simulink library "dsrc_transmitter"  (Simulink 8.2)
settings: Solver=ode1  StartTime=0.0  StopTime=Inf  FixedStep=0.001  RelTol=1e-3
PostLoadFcn:
  | , if any(exist('dsrtsu_mdlpostloadfcn', 'file') == [2, 3, 6]), try dsrtsu_mdlpostloadfcn('Execute', bdroot); catch fprintf('Error in PostLoadFcn (dsrtsu_mdlpostloadfcn) for model "%s":\n %s\n', bdroot, lasterr); end, end,
libraries: simulink x10, rtitttasklib x2, rtiethernetudplib x1, parse_utils x1
(part 1 of 2)
settings Model: DSRTSU_INTERNAL_RTI_VER=440  DSRTSU_INTERNAL_RTI_TYPE=rti1401  DSRTSU_INTERNAL_RTIFPGA=30  Creator=leidos  LastModifiedBy=Admin

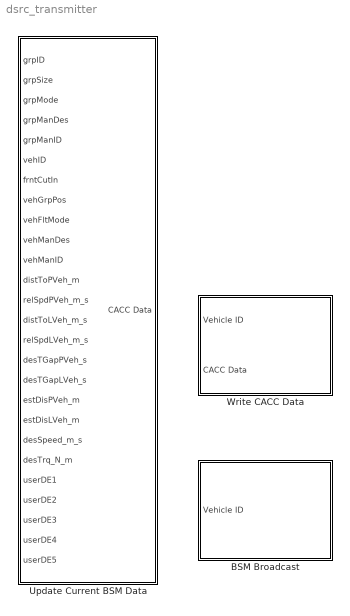
== system dsrc_transmitter ==
  BSM Broadcast : Subsystem
  Update Current BSM Data : Subsystem
  Write CACC Data : Subsystem

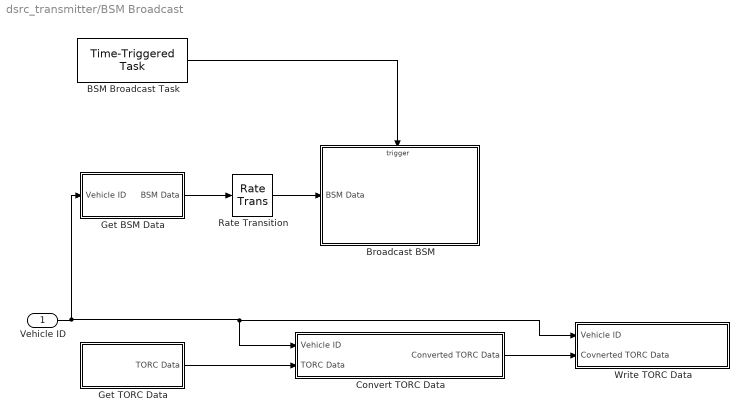
== system dsrc_transmitter/BSM Broadcast ==
  Vehicle ID : Inport
  BSM Broadcast Task : rtitttasklib/Time-Triggered Task  TimeTriggerId=BSM_TX  TLCFileName=rtitimetriggeredtask  DSProperties=struct('RTI',struct('Version',uint32(1),'BlockType',struct('isSLSource',uint8(1),'isSLSink',uint8(0),'isHWSource',uint8(0),'isHWSink',uint8(0),'isSetup',uint8(0),'isInline',uint8(1),'isNonInline',uint8(0),'isInterrupt',uint8(0),'isChannelwise',uint8(0)),'IOBoardType','RTITIMETRIGGER','UnitType','TIMETRIGGERED','Identifier','TASK','DialogType','SL','BlockSet','NONE','SlaveProcessor','NONE'))  RTIBlockInterface=struct('OutputPortsActive',1,'OutputPortsWidth',int32(1),'FunctionCall',uint32(0),'OutputPortsName',{{[' ']}},'InitLevel',3,'BlockDisplay',{{['Time-Triggered Task\nID: ''''BSM_TX'''''],'center'}},'IconTransparency','off','BlockName',struct('Token',{{['Time-Triggered Task']}}),'MaskDescription',['Specifies a time-triggered task. The task trigger times are set by the assigned Time-Trigger Set block.' char(10) '' char(10) 'This block can only be used together with the Time-Trigger Set block.'])  RTIBlockParameters=struct('TimeTriggerId',{{'BSM_TX','OFF',[]}},'TLCFileName',{{'rtitimetriggeredtask','OFF',[]}})  RTISFcnParameters=struct('TLCFileName','char')  RTIBlockParaDefault=struct('TimeTriggerId','TT_ID','TLCFileName','rtitimetriggeredtask')
  Broadcast BSM : Subsystem
  Convert TORC Data : Subsystem
  Get BSM Data : Subsystem
  Get TORC Data : Subsystem
  Rate Transition : RateTransition  Deterministic=off
  Write TORC Data : Subsystem
  wires:
  Get BSM Data/1(BSM Data) -> Rate Transition/1
  BSM Broadcast Task/1 -> Broadcast BSM/Trigger
  Get TORC Data/1(TORC Data) -> Convert TORC Data/2(TORC Data)
  Convert TORC Data/1(Converted TORC Data) -> Write TORC Data/2(Covnerted TORC Data)
  Vehicle ID/1 -> Write TORC Data/1(Vehicle ID), Convert TORC Data/1(Vehicle ID), Get BSM Data/1(Vehicle ID)
  Rate Transition/1 -> Broadcast BSM/1(BSM Data)

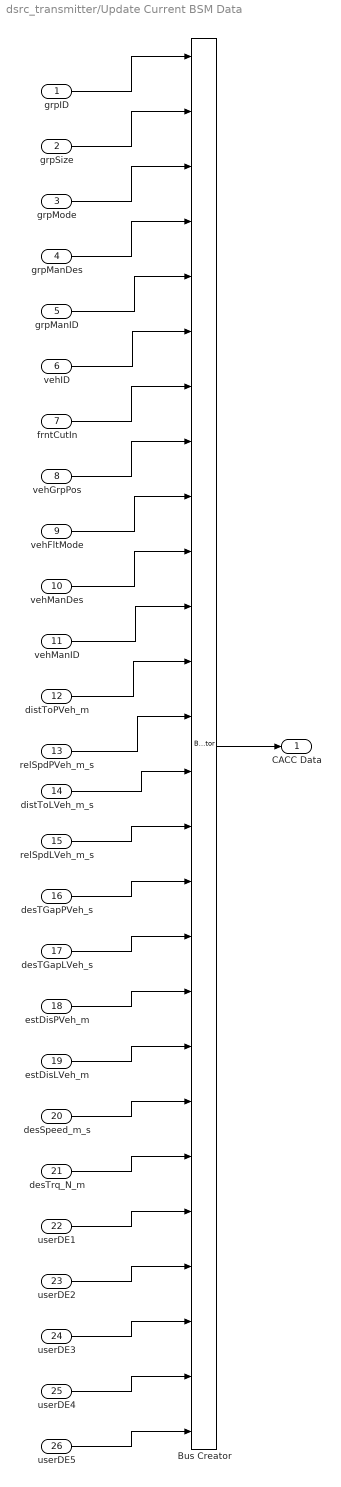
== system dsrc_transmitter/Update Current BSM Data ==
  grpID : Inport
  grpSize : Inport  Port=2
  grpMode : Inport  Port=3
  grpManDes : Inport  Port=4
  grpManID : Inport  Port=5
  vehID : Inport  Port=6
  frntCutIn : Inport  Port=7
  vehGrpPos : Inport  Port=8
  vehFltMode : Inport  Port=9
  vehManDes : Inport  Port=10
  vehManID : Inport  Port=11
  distToPVeh_m : Inport  Port=12
  relSpdPVeh_m_s : Inport  Port=13
  distToLVeh_m_s : Inport  Port=14
  relSpdLVeh_m_s : Inport  Port=15
  desTGapPVeh_s : Inport  Port=16
  desTGapLVeh_s : Inport  Port=17
  estDisPVeh_m : Inport  Port=18
  estDisLVeh_m : Inport  Port=19
  desSpeed_m_s : Inport  Port=20
  desTrq_N_m : Inport  Port=21
  userDE1 : Inport  Port=22
  userDE2 : Inport  Port=23
  userDE3 : Inport  Port=24
  userDE4 : Inport  Port=25
  userDE5 : Inport  Port=26
  Bus Creator : BusCreator  Inputs=26
  CACC Data : Outport
  wires:
  grpID/1 -> Bus Creator/1
  grpSize/1 -> Bus Creator/2
  grpMode/1 -> Bus Creator/3
  grpManDes/1 -> Bus Creator/4
  grpManID/1 -> Bus Creator/5
  vehID/1 -> Bus Creator/6
  frntCutIn/1 -> Bus Creator/7
  vehGrpPos/1 -> Bus Creator/8
  vehFltMode/1 -> Bus Creator/9
  vehManDes/1 -> Bus Creator/10
  vehManID/1 -> Bus Creator/11
  distToPVeh_m/1 -> Bus Creator/12
  relSpdPVeh_m_s/1 -> Bus Creator/13
  distToLVeh_m_s/1 -> Bus Creator/14
  relSpdLVeh_m_s/1 -> Bus Creator/15
  desTGapPVeh_s/1 -> Bus Creator/16
  desTGapLVeh_s/1 -> Bus Creator/17
  estDisPVeh_m/1 -> Bus Creator/18
  estDisLVeh_m/1 -> Bus Creator/19
  desSpeed_m_s/1 -> Bus Creator/20
  desTrq_N_m/1 -> Bus Creator/21
  userDE1/1 -> Bus Creator/22
  userDE2/1 -> Bus Creator/23
  userDE3/1 -> Bus Creator/24
  userDE4/1 -> Bus Creator/25
  userDE5/1 -> Bus Creator/26
  Bus Creator/1 -> CACC Data/1

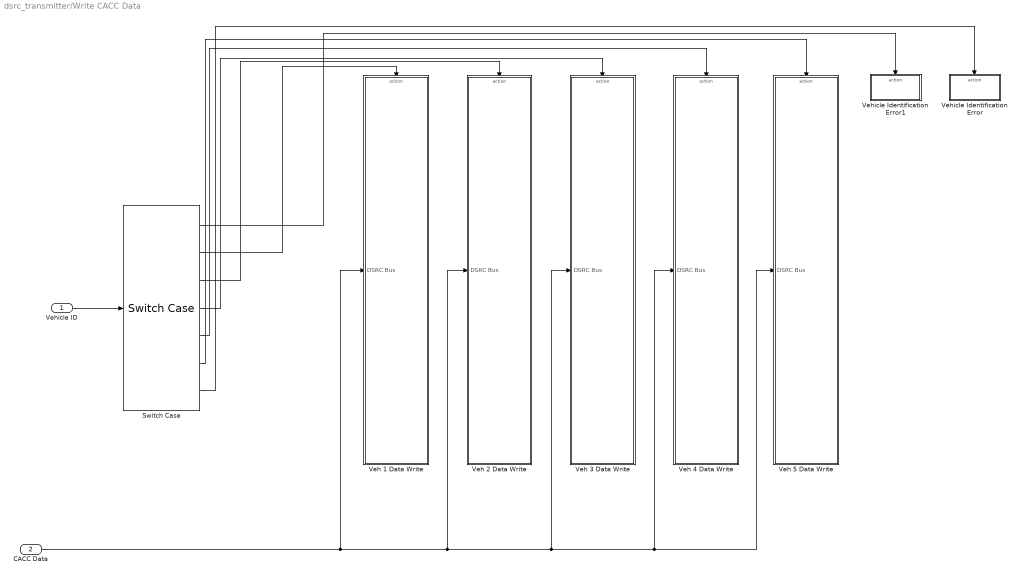
== system dsrc_transmitter/Write CACC Data ==
  Vehicle ID : Inport
  CACC Data : Inport  Port=2
  Switch Case : SwitchCase  CaseConditions={0,96,97,98,99,100}
  Veh 1 Data Write : Subsystem  TreatAsAtomicUnit=on
  Veh 2 Data Write : Subsystem  TreatAsAtomicUnit=on
  Veh 3 Data Write : Subsystem  TreatAsAtomicUnit=on
  Veh 4 Data Write : Subsystem  TreatAsAtomicUnit=on
  Veh 5 Data Write : Subsystem  TreatAsAtomicUnit=on
  Vehicle Identification Error : Subsystem  TreatAsAtomicUnit=on
  Vehicle Identification Error1 : Subsystem  TreatAsAtomicUnit=on
  wires:
  CACC Data/1 -> Veh 5 Data Write/1(DSRC Bus), Veh 4 Data Write/1(DSRC Bus), Veh 3 Data Write/1(DSRC Bus), Veh 2 Data Write/1(DSRC Bus), Veh 1 Data Write/1(DSRC Bus)
  Switch Case/2 -> Veh 1 Data Write/Action
  Switch Case/3 -> Veh 2 Data Write/Action
  Switch Case/4 -> Veh 3 Data Write/Action
  Switch Case/5 -> Veh 4 Data Write/Action
  Switch Case/6 -> Veh 5 Data Write/Action
  Switch Case/1 -> Vehicle Identification Error1/Action
  Switch Case/7 -> Vehicle Identification Error/Action
  Vehicle ID/1 -> Switch Case/1

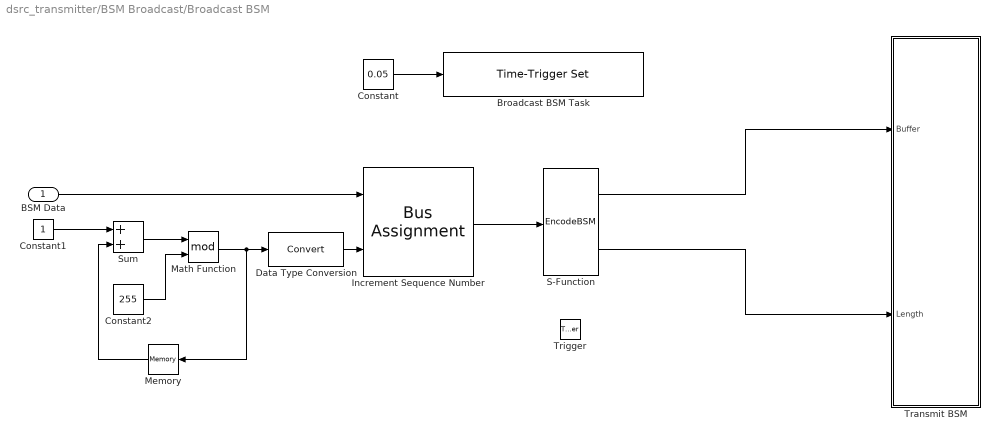
== system dsrc_transmitter/BSM Broadcast/Broadcast BSM ==
  BSM Data : Inport
  Trigger : TriggerPort  TriggerType=function-call  PortDimensions=1
  Broadcast BSM Task : rtitttasklib/Time-Trigger Set  TimeTriggerId=BSM_TX  SampleTime=-1  RegisterAtSimulationStart=on  TLCFileName=rtitimetriggerset  DSProperties=struct('RTI',struct('Version',uint32(1),'BlockType',struct('isSLSource',uint8(1),'isSLSink',uint8(0),'isHWSource',uint8(0),'isHWSink',uint8(0),'isSetup',uint8(0),'isInline',uint8(1),'isNonInline',uint8(0),'isInterrupt',uint8(0),'isChannelwise',uint8(0)),'IOBoardType','RTITIMETRIGGER','UnitType','TIMETRIGGERED','Identifier','SET','DialogType','SL','BlockSet','NONE','SlaveProcessor','NONE'))  RTIBlockInterface=struct('InputPortsActive',1,'InputPortsWidth',{{'DYNAMICALLY_SIZED'}},'InputPortsDataType',{{'SS_DOUBLE'}},'InputPortsName',{{['Trigger delay']}},'InitLevel',3,'BlockDisplay',{{['Time-Trigger Set\nID: ''''BSM_TX'''''],'center'}},'IconTransparency','on','BlockName',struct('Token',{{['Time-Trigger Set']}}),'MaskDescription',['When this block is evaluated it sets the task trigger times for the assigned time-triggered task.' char(10) '' char(10) 'This block can only be used together with the Time-Triggered Task block.'],'SampleTime',{{-1}})  RTIBlockParameters=struct('TimeTriggerId',{{'BSM_TX','OFF',[]}},'SampleTime',{{-1,'OFF',[]}},'RegisterAtSimulationStart',{{logical(1),'OFF',[]}},'TLCFileName',{{'rtitimetriggerset','OFF',[]}})  RTISFcnParameters=struct('TimeTriggerId','char','SampleTime','double','TLCFileName','char','RegisterAtSimulationStart','double')  RTIBlockParaDefault=struct('TimeTriggerId','TT_ID','SampleTime',-1,'RegisterAtSimulationStart',0,'TLCFileName','rtitimetriggerset')
  Constant : Constant  Value=0.05
  Constant1 : Constant
  Constant2 : Constant  Value=255
  Data Type Conversion : DataTypeConversion
  Increment Sequence Number : BusAssignment  AssignedSignals=msgCnt
  Math Function : Math  Operator=mod  SaturateOnIntegerOverflow=on
  Memory : Memory  InheritSampleTime=on
  S-Function : S-Function  FunctionName=EncodeBSM  SFunctionModules='EncodeBSM_wrapper bsm_encoder der_encoder'  EnableBusSupport=off
  Sum : Sum  SaturateOnIntegerOverflow=on  InputSameDT=on  OutDataTypeStr=Inherit: Same as first input
  Transmit BSM : Subsystem
  wires:
  S-Function/1 -> Transmit BSM/1(Buffer)
  S-Function/2 -> Transmit BSM/2(Length)
  BSM Data/1 -> Increment Sequence Number/1
  Constant/1 -> Broadcast BSM Task/1
  Constant1/1 -> Sum/1
  Memory/1 -> Sum/2
  Sum/1 -> Math Function/1
  Increment Sequence Number/1 -> S-Function/1
  Math Function/1 -> Memory/1, Data Type Conversion/1
  Constant2/1 -> Math Function/2
  Data Type Conversion/1 -> Increment Sequence Number/2

== system dsrc_transmitter/BSM Broadcast/Convert TORC Data ==
  Vehicle ID : Inport
  TORC Data : Inport  Port=2
  Data Conversion : Subsystem
  Data Type Conversion : DataTypeConversion
  Converted TORC Data : Outport
  wires:
  TORC Data/1 -> Data Conversion/2(TORC Data)
  Data Conversion/1(BSM Data) -> Converted TORC Data/1
  Vehicle ID/1 -> Data Type Conversion/1
  Data Type Conversion/1 -> Data Conversion/1(Vehicle ID)

== system dsrc_transmitter/BSM Broadcast/Get BSM Data ==
  Vehicle ID : Inport
  BSM Data Read : Subsystem
  BSM Data : Outport
  wires:
  BSM Data Read/1(Cur Veh BSM Data) -> BSM Data/1
  Vehicle ID/1 -> BSM Data Read/1(Veh ID)

== system dsrc_transmitter/BSM Broadcast/Get TORC Data ==
  Bus Creator : BusCreator  Inputs=28
  Data Store Read : DataStoreRead  DataStoreName=CarmaData  DataStoreElements=CarmaData.acc_status#CarmaData.requested_cacc_state#CarmaData.radar_status#CarmaData.throttle_pedal_deflect_percent#CarmaData.acc_set_speed_m_s#CarmaData.local_north_m#CarmaData.local_east_m#CarmaData.local_down_m#CarmaData.global_roll_deg#CarmaData.global_pitch_deg#CarmaData.global_yaw_deg#CarmaData.horizontal_pos_accuracy_m#CarmaData.vertical_pos_accuracy_m#CarmaData.velocity_fwd_m_s#CarmaData.velocity_right_m_s#CarmaData.velocity_down_m_s#CarmaData.velocity_accuracy_m_s#CarmaData.accel_m_s2#CarmaData.accel_right_m_s2#CarmaData.accel_down_m_s2#CarmaData.speed_m_s#CarmaData.steering_wheel_angle_deg#CarmaData.brk_light_flag#CarmaData.global_utc_time_s#CarmaData.global_lat_deg#CarmaData.global_long_deg#CarmaData.global_alt_m#CarmaData.path_ctrl_status.value
  TORC Data : Outport
  wires:
  Data Store Read/1 -> Bus Creator/1
  Data Store Read/2 -> Bus Creator/2
  Data Store Read/3 -> Bus Creator/3
  Data Store Read/4 -> Bus Creator/4
  Data Store Read/5 -> Bus Creator/5
  Data Store Read/6 -> Bus Creator/6
  Data Store Read/7 -> Bus Creator/7
  Data Store Read/8 -> Bus Creator/8
  Data Store Read/9 -> Bus Creator/9
  Data Store Read/10 -> Bus Creator/10
  Data Store Read/12 -> Bus Creator/12
  Data Store Read/13 -> Bus Creator/13
  Data Store Read/14 -> Bus Creator/14
  Data Store Read/15 -> Bus Creator/15
  Data Store Read/16 -> Bus Creator/16
  Data Store Read/17 -> Bus Creator/17
  Data Store Read/18 -> Bus Creator/18
  Data Store Read/19 -> Bus Creator/19
  Data Store Read/20 -> Bus Creator/20
  Data Store Read/21 -> Bus Creator/21
  Data Store Read/22 -> Bus Creator/22
  Data Store Read/23 -> Bus Creator/23
  Data Store Read/11 -> Bus Creator/11
  Bus Creator/1 -> TORC Data/1
  Data Store Read/24 -> Bus Creator/24
  Data Store Read/25 -> Bus Creator/25
  Data Store Read/26 -> Bus Creator/26
  Data Store Read/27 -> Bus Creator/27
  Data Store Read/28 -> Bus Creator/28

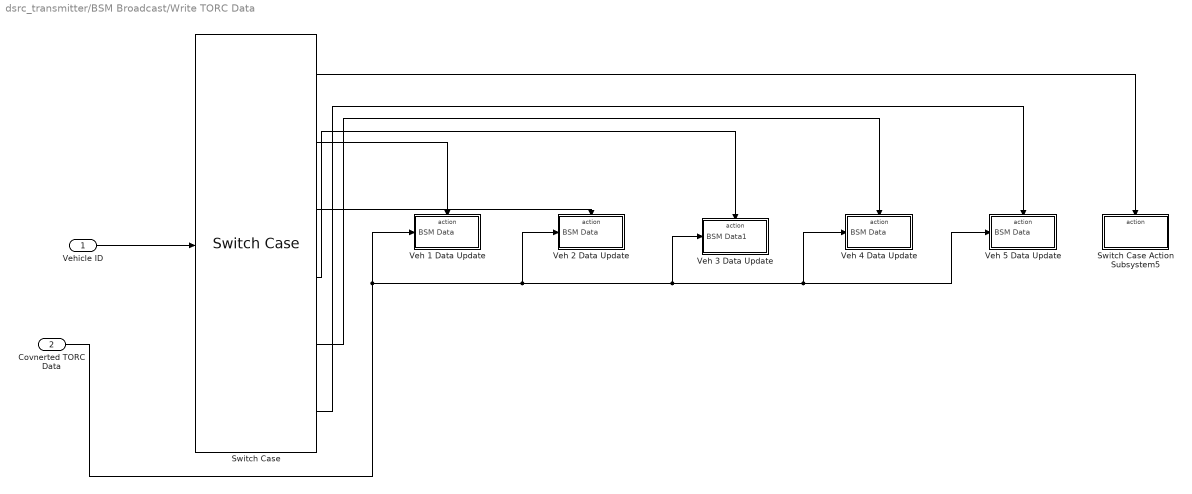
== system dsrc_transmitter/BSM Broadcast/Write TORC Data ==
  Vehicle ID : Inport
  Covnerted TORC Data : Inport  Port=2
  Switch Case : SwitchCase  CaseConditions={0,96,97,98,99,100}  ShowDefaultCase=off
  Switch Case Action Subsystem5 : Subsystem  TreatAsAtomicUnit=on
  Veh 1 Data Update : Subsystem  TreatAsAtomicUnit=on
  Veh 2 Data Update : Subsystem  TreatAsAtomicUnit=on
  Veh 3 Data Update : Subsystem  TreatAsAtomicUnit=on
  Veh 4 Data Update : Subsystem  TreatAsAtomicUnit=on
  Veh 5 Data Update : Subsystem  TreatAsAtomicUnit=on
  wires:
  Switch Case/2 -> Veh 1 Data Update/Action
  Switch Case/3 -> Veh 2 Data Update/Action
  Switch Case/4 -> Veh 3 Data Update/Action
  Switch Case/5 -> Veh 4 Data Update/Action
  Switch Case/6 -> Veh 5 Data Update/Action
  Switch Case/1 -> Switch Case Action Subsystem5/Action
  Covnerted TORC Data/1 -> Veh 1 Data Update/1(BSM Data), Veh 2 Data Update/1(BSM Data), Veh 3 Data Update/1(BSM Data1), Veh 5 Data Update/1(BSM Data), Veh 4 Data Update/1(BSM Data)
  Vehicle ID/1 -> Switch Case/1

== system dsrc_transmitter/Write CACC Data/Veh 1 Data Write ==
  DSRC Bus : Inport
  Action Port : ActionPort
  Bus Selector : BusSelector  OutputSignals=signal1,signal2,signal3,signal4,signal5,signal6,signal7,signal8,signal9,signal10,signal11,signal12,signal13,signal14,signal15,signal16,signal17,signal18,signal19,signal20,signal21,signal22,signal23,signal24,signal25,signal26
  Data Store Write : DataStoreWrite  DataStoreName=BSMStoreSignal  DataStoreElements=BSMStoreSignal.Veh1BSM.grpID#BSMStoreSignal.Veh1BSM.grpSize#BSMStoreSignal.Veh1BSM.grpMode#BSMStoreSignal.Veh1BSM.grpManDes#BSMStoreSignal.Veh1BSM.grpManID#BSMStoreSignal.Veh1BSM.vehID#BSMStoreSignal.Veh1BSM.frntCutIn#BSMStoreSignal.Veh1BSM.vehGrpPos#BSMStoreSignal.Veh1BSM.vehFltMode#BSMStoreSignal.Veh1BSM.vehManDes#BSMStoreSignal.Veh1BSM.vehManID#BSMStoreSignal.Veh1BSM.distToPVeh_m#BSMStoreSignal.Veh1BSM.relSpdPVeh_m_s#BSMStoreSignal.Veh1BSM.distToLVeh_m#BSMStoreSignal.Veh1BSM.relSpdLVeh_m_s#BSMStoreSignal.Veh1BSM.desTGapPVeh_s#BSMStoreSignal.Veh1BSM.desTGapLVeh_s#BSMStoreSignal.Veh1BSM.estDisPVeh_m#BSMStoreSignal.Veh1BSM.estDisLVeh_m#BSMStoreSignal.Veh1BSM.desSpeed_m_s#BSMStoreSignal.Veh1BSM.desTrq_N_m#BSMStoreSignal.Veh1BSM.userDE1#BSMStoreSignal.Veh1BSM.userDE2#BSMStoreSignal.Veh1BSM.userDE3#BSMStoreSignal.Veh1BSM.userDE4#BSMStoreSignal.Veh1BSM.userDE5
  wires:
  DSRC Bus/1 -> Bus Selector/1
  Bus Selector/1 -> Data Store Write/1  "<signal1>"
  Bus Selector/2 -> Data Store Write/2  "<signal2>"
  Bus Selector/3 -> Data Store Write/3  "<signal3>"
  Bus Selector/4 -> Data Store Write/4  "<signal4>"
  Bus Selector/5 -> Data Store Write/5  "<signal5>"
  Bus Selector/6 -> Data Store Write/6  "<signal6>"
  Bus Selector/7 -> Data Store Write/7  "<signal7>"
  Bus Selector/8 -> Data Store Write/8  "<signal8>"
  Bus Selector/9 -> Data Store Write/9  "<signal9>"
  Bus Selector/10 -> Data Store Write/10  "<signal10>"
  Bus Selector/11 -> Data Store Write/11  "<signal11>"
  Bus Selector/12 -> Data Store Write/12  "<signal12>"
  Bus Selector/13 -> Data Store Write/13  "<signal13>"
  Bus Selector/14 -> Data Store Write/14  "<signal14>"
  Bus Selector/15 -> Data Store Write/15  "<signal15>"
  Bus Selector/16 -> Data Store Write/16  "<signal16>"
  Bus Selector/17 -> Data Store Write/17  "<signal17>"
  Bus Selector/18 -> Data Store Write/18  "<signal18>"
  Bus Selector/19 -> Data Store Write/19  "<signal19>"
  Bus Selector/20 -> Data Store Write/20  "<signal20>"
  Bus Selector/21 -> Data Store Write/21  "<signal21>"
  Bus Selector/22 -> Data Store Write/22  "<signal22>"
  Bus Selector/23 -> Data Store Write/23  "<signal23>"
  Bus Selector/24 -> Data Store Write/24  "<signal24>"
  Bus Selector/25 -> Data Store Write/25  "<signal25>"
  Bus Selector/26 -> Data Store Write/26  "<signal26>"

== system dsrc_transmitter/Write CACC Data/Veh 2 Data Write ==
  DSRC Bus : Inport
  Action Port : ActionPort
  Bus Selector : BusSelector  OutputSignals=signal1,signal2,signal3,signal4,signal5,signal6,signal7,signal8,signal9,signal10,signal11,signal12,signal13,signal14,signal15,signal16,signal17,signal18,signal19,signal20,signal21,signal22,signal23,signal24,signal25,signal26
  Data Store Write : DataStoreWrite  DataStoreName=BSMStoreSignal  DataStoreElements=BSMStoreSignal.Veh2BSM.grpID#BSMStoreSignal.Veh2BSM.grpSize#BSMStoreSignal.Veh2BSM.grpMode#BSMStoreSignal.Veh2BSM.grpManDes#BSMStoreSignal.Veh2BSM.grpManID#BSMStoreSignal.Veh2BSM.vehID#BSMStoreSignal.Veh2BSM.frntCutIn#BSMStoreSignal.Veh2BSM.vehGrpPos#BSMStoreSignal.Veh2BSM.vehFltMode#BSMStoreSignal.Veh2BSM.vehManDes#BSMStoreSignal.Veh2BSM.vehManID#BSMStoreSignal.Veh2BSM.distToPVeh_m#BSMStoreSignal.Veh2BSM.relSpdPVeh_m_s#BSMStoreSignal.Veh2BSM.distToLVeh_m#BSMStoreSignal.Veh2BSM.relSpdLVeh_m_s#BSMStoreSignal.Veh2BSM.desTGapPVeh_s#BSMStoreSignal.Veh2BSM.desTGapLVeh_s#BSMStoreSignal.Veh2BSM.estDisPVeh_m#BSMStoreSignal.Veh2BSM.estDisLVeh_m#BSMStoreSignal.Veh2BSM.desSpeed_m_s#BSMStoreSignal.Veh2BSM.desTrq_N_m#BSMStoreSignal.Veh2BSM.userDE1#BSMStoreSignal.Veh2BSM.userDE2#BSMStoreSignal.Veh2BSM.userDE3#BSMStoreSignal.Veh2BSM.userDE4#BSMStoreSignal.Veh2BSM.userDE5
  wires:
  DSRC Bus/1 -> Bus Selector/1
  Bus Selector/1 -> Data Store Write/1  "<signal1>"
  Bus Selector/2 -> Data Store Write/2  "<signal2>"
  Bus Selector/3 -> Data Store Write/3  "<signal3>"
  Bus Selector/4 -> Data Store Write/4  "<signal4>"
  Bus Selector/5 -> Data Store Write/5  "<signal5>"
  Bus Selector/6 -> Data Store Write/6  "<signal6>"
  Bus Selector/7 -> Data Store Write/7  "<signal7>"
  Bus Selector/8 -> Data Store Write/8  "<signal8>"
  Bus Selector/9 -> Data Store Write/9  "<signal9>"
  Bus Selector/10 -> Data Store Write/10  "<signal10>"
  Bus Selector/11 -> Data Store Write/11  "<signal11>"
  Bus Selector/12 -> Data Store Write/12  "<signal12>"
  Bus Selector/13 -> Data Store Write/13  "<signal13>"
  Bus Selector/14 -> Data Store Write/14  "<signal14>"
  Bus Selector/15 -> Data Store Write/15  "<signal15>"
  Bus Selector/16 -> Data Store Write/16  "<signal16>"
  Bus Selector/17 -> Data Store Write/17  "<signal17>"
  Bus Selector/18 -> Data Store Write/18  "<signal18>"
  Bus Selector/19 -> Data Store Write/19  "<signal19>"
  Bus Selector/20 -> Data Store Write/20  "<signal20>"
  Bus Selector/21 -> Data Store Write/21  "<signal21>"
  Bus Selector/22 -> Data Store Write/22  "<signal22>"
  Bus Selector/23 -> Data Store Write/23  "<signal23>"
  Bus Selector/24 -> Data Store Write/24  "<signal24>"
  Bus Selector/25 -> Data Store Write/25  "<signal25>"
  Bus Selector/26 -> Data Store Write/26  "<signal26>"

== system dsrc_transmitter/Write CACC Data/Veh 3 Data Write ==
  DSRC Bus : Inport
  Action Port : ActionPort
  Bus Selector : BusSelector  OutputSignals=signal1,signal2,signal3,signal4,signal5,signal6,signal7,signal8,signal9,signal10,signal11,signal12,signal13,signal14,signal15,signal16,signal17,signal18,signal19,signal20,signal21,signal22,signal23,signal24,signal25,signal26
  Data Store Write : DataStoreWrite  DataStoreName=BSMStoreSignal  DataStoreElements=BSMStoreSignal.Veh3BSM.grpID#BSMStoreSignal.Veh3BSM.grpSize#BSMStoreSignal.Veh3BSM.grpMode#BSMStoreSignal.Veh3BSM.grpManDes#BSMStoreSignal.Veh3BSM.grpManID#BSMStoreSignal.Veh3BSM.vehID#BSMStoreSignal.Veh3BSM.frntCutIn#BSMStoreSignal.Veh3BSM.vehGrpPos#BSMStoreSignal.Veh3BSM.vehFltMode#BSMStoreSignal.Veh3BSM.vehManDes#BSMStoreSignal.Veh3BSM.vehManID#BSMStoreSignal.Veh3BSM.distToPVeh_m#BSMStoreSignal.Veh3BSM.relSpdPVeh_m_s#BSMStoreSignal.Veh3BSM.distToLVeh_m#BSMStoreSignal.Veh3BSM.relSpdLVeh_m_s#BSMStoreSignal.Veh3BSM.desTGapPVeh_s#BSMStoreSignal.Veh3BSM.desTGapLVeh_s#BSMStoreSignal.Veh3BSM.estDisPVeh_m#BSMStoreSignal.Veh3BSM.estDisLVeh_m#BSMStoreSignal.Veh3BSM.desSpeed_m_s#BSMStoreSignal.Veh3BSM.desTrq_N_m#BSMStoreSignal.Veh3BSM.userDE1#BSMStoreSignal.Veh3BSM.userDE2#BSMStoreSignal.Veh3BSM.userDE3#BSMStoreSignal.Veh3BSM.userDE4#BSMStoreSignal.Veh3BSM.userDE5
  wires:
  DSRC Bus/1 -> Bus Selector/1
  Bus Selector/1 -> Data Store Write/1  "<signal1>"
  Bus Selector/2 -> Data Store Write/2  "<signal2>"
  Bus Selector/3 -> Data Store Write/3  "<signal3>"
  Bus Selector/4 -> Data Store Write/4  "<signal4>"
  Bus Selector/5 -> Data Store Write/5  "<signal5>"
  Bus Selector/6 -> Data Store Write/6  "<signal6>"
  Bus Selector/7 -> Data Store Write/7  "<signal7>"
  Bus Selector/8 -> Data Store Write/8  "<signal8>"
  Bus Selector/9 -> Data Store Write/9  "<signal9>"
  Bus Selector/10 -> Data Store Write/10  "<signal10>"
  Bus Selector/11 -> Data Store Write/11  "<signal11>"
  Bus Selector/12 -> Data Store Write/12  "<signal12>"
  Bus Selector/13 -> Data Store Write/13  "<signal13>"
  Bus Selector/14 -> Data Store Write/14  "<signal14>"
  Bus Selector/15 -> Data Store Write/15  "<signal15>"
  Bus Selector/16 -> Data Store Write/16  "<signal16>"
  Bus Selector/17 -> Data Store Write/17  "<signal17>"
  Bus Selector/18 -> Data Store Write/18  "<signal18>"
  Bus Selector/19 -> Data Store Write/19  "<signal19>"
  Bus Selector/20 -> Data Store Write/20  "<signal20>"
  Bus Selector/21 -> Data Store Write/21  "<signal21>"
  Bus Selector/22 -> Data Store Write/22  "<signal22>"
  Bus Selector/23 -> Data Store Write/23  "<signal23>"
  Bus Selector/24 -> Data Store Write/24  "<signal24>"
  Bus Selector/25 -> Data Store Write/25  "<signal25>"
  Bus Selector/26 -> Data Store Write/26  "<signal26>"

== system dsrc_transmitter/Write CACC Data/Veh 4 Data Write ==
  DSRC Bus : Inport
  Action Port : ActionPort
  Bus Selector : BusSelector  OutputSignals=signal1,signal2,signal3,signal4,signal5,signal6,signal7,signal8,signal9,signal10,signal11,signal12,signal13,signal14,signal15,signal16,signal17,signal18,signal19,signal20,signal21,signal22,signal23,signal24,signal25,signal26
  Data Store Write : DataStoreWrite  DataStoreName=BSMStoreSignal  DataStoreElements=BSMStoreSignal.Veh4BSM.grpID#BSMStoreSignal.Veh4BSM.grpSize#BSMStoreSignal.Veh4BSM.grpMode#BSMStoreSignal.Veh4BSM.grpManDes#BSMStoreSignal.Veh4BSM.grpManID#BSMStoreSignal.Veh4BSM.vehID#BSMStoreSignal.Veh4BSM.frntCutIn#BSMStoreSignal.Veh4BSM.vehGrpPos#BSMStoreSignal.Veh4BSM.vehFltMode#BSMStoreSignal.Veh4BSM.vehManDes#BSMStoreSignal.Veh4BSM.vehManID#BSMStoreSignal.Veh4BSM.distToPVeh_m#BSMStoreSignal.Veh4BSM.relSpdPVeh_m_s#BSMStoreSignal.Veh4BSM.distToLVeh_m#BSMStoreSignal.Veh4BSM.relSpdLVeh_m_s#BSMStoreSignal.Veh4BSM.desTGapPVeh_s#BSMStoreSignal.Veh4BSM.desTGapLVeh_s#BSMStoreSignal.Veh4BSM.estDisPVeh_m#BSMStoreSignal.Veh4BSM.estDisLVeh_m#BSMStoreSignal.Veh4BSM.desSpeed_m_s#BSMStoreSignal.Veh4BSM.desTrq_N_m#BSMStoreSignal.Veh4BSM.userDE1#BSMStoreSignal.Veh4BSM.userDE2#BSMStoreSignal.Veh4BSM.userDE3#BSMStoreSignal.Veh4BSM.userDE4#BSMStoreSignal.Veh4BSM.userDE5
  wires:
  DSRC Bus/1 -> Bus Selector/1
  Bus Selector/1 -> Data Store Write/1  "<signal1>"
  Bus Selector/2 -> Data Store Write/2  "<signal2>"
  Bus Selector/3 -> Data Store Write/3  "<signal3>"
  Bus Selector/4 -> Data Store Write/4  "<signal4>"
  Bus Selector/5 -> Data Store Write/5  "<signal5>"
  Bus Selector/6 -> Data Store Write/6  "<signal6>"
  Bus Selector/7 -> Data Store Write/7  "<signal7>"
  Bus Selector/8 -> Data Store Write/8  "<signal8>"
  Bus Selector/9 -> Data Store Write/9  "<signal9>"
  Bus Selector/10 -> Data Store Write/10  "<signal10>"
  Bus Selector/11 -> Data Store Write/11  "<signal11>"
  Bus Selector/12 -> Data Store Write/12  "<signal12>"
  Bus Selector/13 -> Data Store Write/13  "<signal13>"
  Bus Selector/14 -> Data Store Write/14  "<signal14>"
  Bus Selector/15 -> Data Store Write/15  "<signal15>"
  Bus Selector/16 -> Data Store Write/16  "<signal16>"
  Bus Selector/17 -> Data Store Write/17  "<signal17>"
  Bus Selector/18 -> Data Store Write/18  "<signal18>"
  Bus Selector/19 -> Data Store Write/19  "<signal19>"
  Bus Selector/20 -> Data Store Write/20  "<signal20>"
  Bus Selector/21 -> Data Store Write/21  "<signal21>"
  Bus Selector/22 -> Data Store Write/22  "<signal22>"
  Bus Selector/23 -> Data Store Write/23  "<signal23>"
  Bus Selector/24 -> Data Store Write/24  "<signal24>"
  Bus Selector/25 -> Data Store Write/25  "<signal25>"
  Bus Selector/26 -> Data Store Write/26  "<signal26>"

== system dsrc_transmitter/Write CACC Data/Veh 5 Data Write ==
  DSRC Bus : Inport
  Action Port : ActionPort
  Bus Selector : BusSelector  OutputSignals=signal1,signal2,signal3,signal4,signal5,signal6,signal7,signal8,signal9,signal10,signal11,signal12,signal13,signal14,signal15,signal16,signal17,signal18,signal19,signal20,signal21,signal22,signal23,signal24,signal25,signal26
  Data Store Write : DataStoreWrite  DataStoreName=BSMStoreSignal  DataStoreElements=BSMStoreSignal.Veh5BSM.grpID#BSMStoreSignal.Veh5BSM.grpSize#BSMStoreSignal.Veh5BSM.grpMode#BSMStoreSignal.Veh5BSM.grpManDes#BSMStoreSignal.Veh5BSM.grpManID#BSMStoreSignal.Veh5BSM.vehID#BSMStoreSignal.Veh5BSM.frntCutIn#BSMStoreSignal.Veh5BSM.vehGrpPos#BSMStoreSignal.Veh5BSM.vehFltMode#BSMStoreSignal.Veh5BSM.vehManDes#BSMStoreSignal.Veh5BSM.vehManID#BSMStoreSignal.Veh5BSM.distToPVeh_m#BSMStoreSignal.Veh5BSM.relSpdPVeh_m_s#BSMStoreSignal.Veh5BSM.distToLVeh_m#BSMStoreSignal.Veh5BSM.relSpdLVeh_m_s#BSMStoreSignal.Veh5BSM.desTGapPVeh_s#BSMStoreSignal.Veh5BSM.desTGapLVeh_s#BSMStoreSignal.Veh5BSM.estDisPVeh_m#BSMStoreSignal.Veh5BSM.estDisLVeh_m#BSMStoreSignal.Veh5BSM.desSpeed_m_s#BSMStoreSignal.Veh5BSM.desTrq_N_m#BSMStoreSignal.Veh5BSM.userDE1#BSMStoreSignal.Veh5BSM.userDE2#BSMStoreSignal.Veh5BSM.userDE3#BSMStoreSignal.Veh5BSM.userDE4#BSMStoreSignal.Veh5BSM.userDE5
  wires:
  DSRC Bus/1 -> Bus Selector/1
  Bus Selector/1 -> Data Store Write/1  "<signal1>"
  Bus Selector/2 -> Data Store Write/2  "<signal2>"
  Bus Selector/3 -> Data Store Write/3  "<signal3>"
  Bus Selector/4 -> Data Store Write/4  "<signal4>"
  Bus Selector/5 -> Data Store Write/5  "<signal5>"
  Bus Selector/6 -> Data Store Write/6  "<signal6>"
  Bus Selector/7 -> Data Store Write/7  "<signal7>"
  Bus Selector/8 -> Data Store Write/8  "<signal8>"
  Bus Selector/9 -> Data Store Write/9  "<signal9>"
  Bus Selector/10 -> Data Store Write/10  "<signal10>"
  Bus Selector/11 -> Data Store Write/11  "<signal11>"
  Bus Selector/12 -> Data Store Write/12  "<signal12>"
  Bus Selector/13 -> Data Store Write/13  "<signal13>"
  Bus Selector/14 -> Data Store Write/14  "<signal14>"
  Bus Selector/15 -> Data Store Write/15  "<signal15>"
  Bus Selector/16 -> Data Store Write/16  "<signal16>"
  Bus Selector/17 -> Data Store Write/17  "<signal17>"
  Bus Selector/18 -> Data Store Write/18  "<signal18>"
  Bus Selector/19 -> Data Store Write/19  "<signal19>"
  Bus Selector/20 -> Data Store Write/20  "<signal20>"
  Bus Selector/21 -> Data Store Write/21  "<signal21>"
  Bus Selector/22 -> Data Store Write/22  "<signal22>"
  Bus Selector/23 -> Data Store Write/23  "<signal23>"
  Bus Selector/24 -> Data Store Write/24  "<signal24>"
  Bus Selector/25 -> Data Store Write/25  "<signal25>"
  Bus Selector/26 -> Data Store Write/26  "<signal26>"

== system dsrc_transmitter/Write CACC Data/Vehicle Identification Error ==
  note: Error Handling Goes Here
  Action Port : ActionPort

== system dsrc_transmitter/Write CACC Data/Vehicle Identification Error1 ==
  note: Error Handling Goes Here
  Action Port : ActionPort

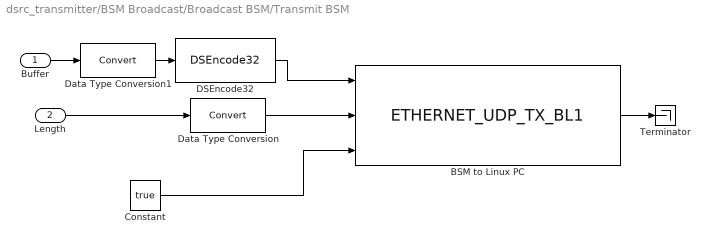
== system dsrc_transmitter/BSM Broadcast/Broadcast BSM/Transmit BSM ==
  Buffer : Inport
  Length : Inport  Port=2
  BSM to Linux PC : rtiethernetudplib/ETHERNET_UDP_TX_BL1  InterfaceName=rti_ethernet_interface_name  BoardType=ETH Type 1  ModuleNo=1  ChannelNo=1  SocketNo=2  MaxMessageSize=1472  SendTimeout=0.0005  LocalSocket=192.168.88.21:5001  RemoteSocket=192.168.88.10:5001  DSProperties=struct('RTI',struct('Version',uint32(2),'BlockType',struct('isSLSource',uint8(1),'isSLSink',uint8(1),'isHWSource',uint8(1),'isHWSink',uint8(1),'isSetup',uint8(0),'isInline',uint8(1),'isNonInline',uint8(1),'isInterrupt',uint8(0),'isChannelwise',uint8(1)),'IOBoardType','DSETHERNETUDP','UnitType','ETHUDP','Identifier','TX','DialogType','SL','BlockSet','RTIETHERNETUDP','SlaveProcessor','NONE'))  RTIBlockInterface=struct('OutputPortsWidth',int32(1),'OutputPortsActive',1,'OutputPortsName',{{'Status'}},'OutputPortsDataType',{{'SS_UINT16'}},'InputPortsWidth',int32([1 1 1]),'InputPortsActive',[1 1 1],'InputPortsName',{{'Data',['Message Size'],'Enable'}},'InputPortsDataType',{{'SS_UINT32','SS_INT32','SS_BOOLEAN'}},'BlockDisplay',{{['Ethernet UDP Transmit\nBoard Type: ETH Type 1\nModule: 1\nSocket: 2\nMaximum Message Size: 1472'],'center'}},'IconTransparency','on','InitLevel',3,'BlockName',struct('Token',{{'ETHERNET_UDP_TX_BL1'}}),'MaskDescription',['To send messages via the Ethernet UDP interface.'])  RTIBlockParameters=struct('InterfaceName',{{'rti_ethernet_interface_name','OFF',[]}},'BoardType',{{1,'OFF',[]}},'ModuleNo',{{1,'OFF',[1 16]}},'ChannelNo',{{1,'OFF',[1 2]}},'SocketNo',{{2,'OFF',[1 4]}},'MaxMessageSize',{{1472,'ON',[1 1472]}},'SendTimeout',{{0.0005,'ON',[1e-05 2]}},'LocalSocket',{{'192.168.88.21:5001','OFF',[]}},'RemoteSocket',{{'192.168.88.10:5001','OFF',[]}})  RTISFcnParameters=struct('InterfaceName','char','BoardType','double','ModuleNo','double','ChannelNo','double','SocketNo','double','MaxMessageSize','double','SendTimeout','double','LocalSocket','char','RemoteSocket','char')  RTIBlockParaDefault=struct('InterfaceName','rti_ethernet_interface_name','BoardType',1,'ModuleNo',1,'ChannelNo',1,'SocketNo',1,'MaxMessageSize',625,'SendTimeout',0.0005,'LocalSocket','XXX.XXX.XXX.XXX:5000','RemoteSocket','XXX.XXX.XXX.XXX:5000')
  Constant : Constant  Value=true
  DSEncode32 : parse_utils/DSEncode32  byteordering=big endian (Motorola)  offset=[ 0 ]  auto_offset=on  datatype=3  one_datatype=on  sampletime=-1
  Data Type Conversion : DataTypeConversion
  Data Type Conversion1 : DataTypeConversion
  Terminator : Terminator
  wires:
  Length/1 -> Data Type Conversion/1
  Constant/1 -> BSM to Linux PC/3
  BSM to Linux PC/1 -> Terminator/1
  DSEncode32/1 -> BSM to Linux PC/1
  Buffer/1 -> Data Type Conversion1/1
  Data Type Conversion/1 -> BSM to Linux PC/2
  Data Type Conversion1/1 -> DSEncode32/1

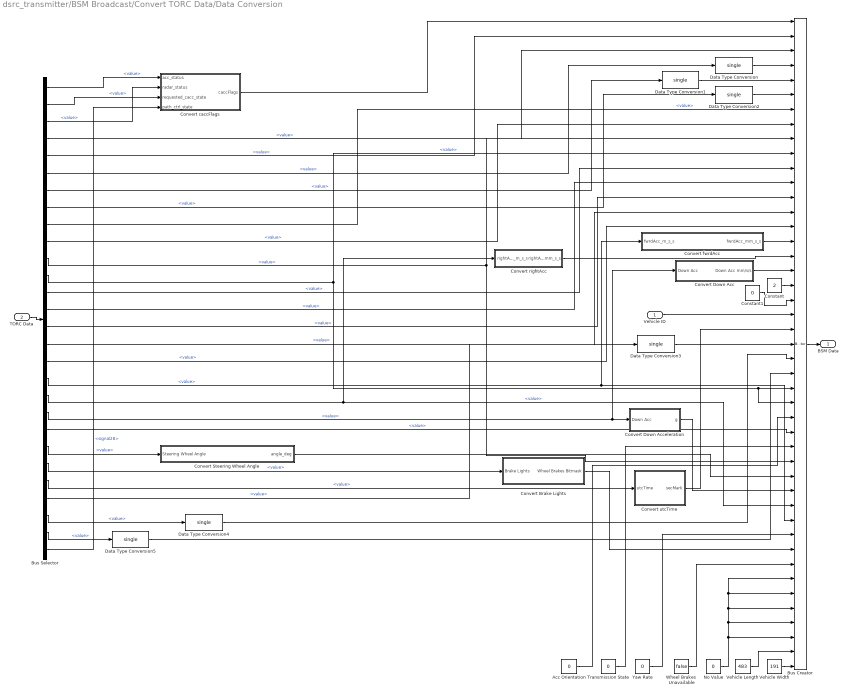
== system dsrc_transmitter/BSM Broadcast/Convert TORC Data/Data Conversion ==
  Vehicle ID : Inport
  TORC Data : Inport  Port=2
  Acc Orientation : Constant  Value=0  OutDataTypeStr=Inherit: Inherit via back propagation
  Bus Creator : BusCreator  Inputs=45
  Bus Selector : BusSelector  OutputSignals=signal1.value,signal2.value,signal3.value,signal4.value,signal5.value,signal6.value,signal7.value,signal8.value,signal9.value,signal10.value,signal11.value,signal12.value,signal13.value,signal14.value,signal15.value,signal16.value,signal17.value,signal18.value,signal19.value,signal20.value,signal21.value,signal22.value,signal23.value,signal24.value,signal25.value,signal26.value,signal27.value,signal28
  Constant : Constant  Value=2  OutDataTypeStr=Inherit: Inherit via back propagation
  Constant1 : Constant  Value=0  OutDataTypeStr=Inherit: Inherit via back propagation
  Convert Brake Lights : Subsystem
  Convert Down Acc : Subsystem
  Convert Down Acceleration : Subsystem
  Convert Steering Wheel Angle : Subsystem
  Convert caccFlags : Subsystem
  Convert fwrdAcc : Subsystem
  Convert rightAcc : Subsystem
  Convert utcTime : Subsystem
  Data Type Conversion{,1..5} (6 alike) : DataTypeConversion  OutDataTypeStr=single
  No Value : Constant  Value=0  OutDataTypeStr=Inherit: Inherit via back propagation
  Transmission State : Constant  Value=0  OutDataTypeStr=Inherit: Inherit via back propagation
  Vehicle Length : Constant  Value=483  OutDataTypeStr=Inherit: Inherit via back propagation
  Vehicle Width : Constant  Value=191  OutDataTypeStr=Inherit: Inherit via back propagation
  Wheel Brakes  Unavailable : Constant  Value=false
  Yaw Rate : Constant  Value=0  OutDataTypeStr=Inherit: Inherit via back propagation
  BSM Data : Outport
  wires:
  Bus Creator/1 -> BSM Data/1
  TORC Data/1 -> Bus Selector/1
  Bus Selector/1 -> Convert caccFlags/1(acc_status)  "<value>"
  Bus Selector/2 -> Convert caccFlags/3(requested_cacc_state)  "<value>"
  Bus Selector/3 -> Convert caccFlags/2(radar_status)  "<value>"
  Convert caccFlags/1(caccFlags) -> Bus Creator/1
  Bus Selector/4 -> Bus Creator/3  "<value>"
  Bus Selector/5 -> Bus Creator/2  "<value>"
  Bus Selector/6 -> Data Type Conversion/1  "<value>"
  Bus Selector/7 -> Data Type Conversion1/1  "<value>"
  Bus Selector/8 -> Data Type Conversion2/1  "<value>"
  Bus Selector/9 -> Bus Creator/7  "<value>"
  Bus Selector/10 -> Bus Creator/8  "<value>"
  Bus Selector/11 -> Bus Creator/9, Bus Creator/31  "<value>"
  Bus Selector/12 -> Bus Creator/27, Bus Creator/26, Bus Creator/10  "<value>"
  Bus Selector/13 -> Bus Creator/11  "<value>"
  Bus Selector/14 -> Bus Creator/12  "<value>"
  Bus Selector/15 -> Bus Creator/13  "<value>"
  Bus Selector/16 -> Bus Creator/14  "<value>"
  Bus Selector/17 -> Bus Creator/15  "<value>"
  Bus Selector/18 -> Convert fwrdAcc/1(fwrdAcc_m_s_s), Bus Creator/35  "<value>"
  Bus Selector/19 -> Bus Creator/34, Convert rightAcc/1(rightAcc_m_s_s)  "<value>"
  Bus Selector/20 -> Convert Down Acceleration/1(Down Acc), Convert Down Acc/1(Down Acc)  "<value>"
  Constant/1 -> Bus Creator/19
  Constant1/1 -> Bus Creator/20
  Vehicle ID/1 -> Bus Creator/21
  Bus Selector/24 -> Convert utcTime/1(utcTime)  "<value>"
  Convert utcTime/1(secMark) -> Bus Creator/22
  Bus Selector/25 -> Data Type Conversion3/1  "<value>"
  Bus Selector/26 -> Data Type Conversion4/1  "<value>"
  Bus Selector/27 -> Data Type Conversion5/1  "<value>"
  Bus Selector/23 -> Convert Brake Lights/1(Brake Lights)  "<value>"
  Convert Brake Lights/1(Wheel Brakes Bitmask) -> Bus Creator/37
  Bus Selector/22 -> Convert Steering Wheel Angle/1(Steering Wheel Angle)  "<value>"
  Convert Steering Wheel Angle/1(angle_deg) -> Bus Creator/32
  Bus Selector/21 -> Bus Creator/29  "<value>"
  Vehicle Width/1 -> Bus Creator/45
  Vehicle Length/1 -> Bus Creator/44
  No Value/1 -> Bus Creator/43, Bus Creator/42, Bus Creator/41, Bus Creator/39, Bus Creator/40
  Wheel Brakes  Unavailable/1 -> Bus Creator/38
  Yaw Rate/1 -> Bus Creator/36
  Convert Down Acceleration/1(g) -> Bus Creator/33
  Convert Down Acc/1(Down Acc mm/s/s) -> Bus Creator/18
  Transmission State/1 -> Bus Creator/30
  Acc Orientation/1 -> Bus Creator/28
  Data Type Conversion/1 -> Bus Creator/4
  Data Type Conversion1/1 -> Bus Creator/5
  Data Type Conversion2/1 -> Bus Creator/6
  Convert fwrdAcc/1(fwrdAcc_mm_s_s) -> Bus Creator/16
  Convert rightAcc/1(rightAcc_mm_s_s) -> Bus Creator/17
  Data Type Conversion3/1 -> Bus Creator/23
  Data Type Conversion4/1 -> Bus Creator/24
  Data Type Conversion5/1 -> Bus Creator/25
  Bus Selector/28 -> Convert caccFlags/4(path_ctrl_state)  "<signal28>"

== system dsrc_transmitter/BSM Broadcast/Get BSM Data/BSM Data Read ==
  Veh ID : Inport
  Get BSM Data : Subsystem
  Cur Veh BSM Data : Outport
  wires:
  Veh ID/1 -> Get BSM Data/1(Veh ID)
  Get BSM Data/1(BSM Data) -> Cur Veh BSM Data/1

== system dsrc_transmitter/BSM Broadcast/Write TORC Data/Switch Case Action Subsystem5 ==
  note: Error Handling Logic Goes Here
  Action Port : ActionPort

== system dsrc_transmitter/BSM Broadcast/Write TORC Data/Veh 1 Data Update ==
  BSM Data : Inport
  Action Port : ActionPort
  Bus Selector : BusSelector  OutputSignals=signal1 (signal 1),value (signal 2),value (signal 3),signal4 (signal 4),signal5 (signal 5),signal6 (signal 6),value (signal 7),value (signal 8),value (signal 9),value (signal 10),value (signal 11),value (signal 12),value (signal 13),value (signal 14),value (signal 15),signal16 (signal 16),signal17 (signal 17),signal18 (signal 18),signal19 (signal 19),signal20 (signal 20),signal21 (signal 21),signal22 (signal 22),signal23 (signal 23),signal24 (signal 24),signal25 (signal 25),value (signal 26),value (signal 27),signal28 (signal 28),value (signal 29),signal30 (signal 30),value (signal 31),signal32 (signal 32),signal33 (signal 33),value (signal 34),value (signal 35),signal36 (signal 36),signal37 (signal 37),signal38 (signal 38),signal39 (signal 39),signal40 (signal 40),signal41 (signal 41),signal42 (signal 42),signal43 (signal 43),signal44 (signal 44),signal45 (signal 45)
  Data Store Write : DataStoreWrite  DataStoreName=BSMStoreSignal  DataStoreElements=BSMStoreSignal.Veh1BSM.caccFlags_bitmask#BSMStoreSignal.Veh1BSM.setSpeed_m_s#BSMStoreSignal.Veh1BSM.throtPos_percent#BSMStoreSignal.Veh1BSM.lclPN_mm#BSMStoreSignal.Veh1BSM.lclPE_mm#BSMStoreSignal.Veh1BSM.lclPD_mm#BSMStoreSignal.Veh1BSM.roll_deg#BSMStoreSignal.Veh1BSM.pitch_deg#BSMStoreSignal.Veh1BSM.yaw_deg#BSMStoreSignal.Veh1BSM.hPosAcry_m#BSMStoreSignal.Veh1BSM.vPosAcry_m#BSMStoreSignal.Veh1BSM.frwdVel_m_s#BSMStoreSignal.Veh1BSM.rightVel_m_s#BSMStoreSignal.Veh1BSM.downVel_m_s#BSMStoreSignal.Veh1BSM.velAcc_m_s#BSMStoreSignal.Veh1BSM.frwdAcc_mm_s_s#BSMStoreSignal.Veh1BSM.rightAcc_mm_s_s#BSMStoreSignal.Veh1BSM.dwnAcc_mm_s_s#BSMStoreSignal.Veh1BSM.msgID#BSMStoreSignal.Veh1BSM.msgCnt#BSMStoreSignal.Veh1BSM.id#BSMStoreSignal.Veh1BSM.secMark_ms#BSMStoreSignal.Veh1BSM.lat_deg#BSMStoreSignal.Veh1BSM.lon_deg#BSMStoreSignal.Veh1BSM.elev_m#BSMStoreSignal.Veh1BSM.semi_major_accuracy_m#BSMStoreSignal.Veh1BSM.semi_minor_accuracy_m#BSMStoreSignal.Veh1BSM.semi_major_accuracy_orientation_deg#BSMStoreSignal.Veh1BSM.speed_m_s#BSMStoreSignal.Veh1BSM.transmission_enum#BSMStoreSignal.Veh1BSM.heading_deg#BSMStoreSignal.Veh1BSM.angle_deg#BSMStoreSignal.Veh1BSM.vertical_acceleration_g#BSMStoreSignal.Veh1BSM.lat_acceleration_m_s_s#BSMStoreSignal.Veh1BSM.long_acceleration_m_s_s#BSMStoreSignal.Veh1BSM.yaw_rate_deg_s#BSMStoreSignal.Veh1BSM.wheelBrakes_bitmask#BSMStoreSignal.Veh1BSM.wheelBrakesUnavailable#BSMStoreSignal.Veh1BSM.tractionControlState_enum#BSMStoreSignal.Veh1BSM.anti_lock_brake_status_enum#BSMStoreSignal.Veh1BSM.stability_control_status_enum#BSMStoreSignal.Veh1BSM.brake_boost_enum#BSMStoreSignal.Veh1BSM.auxiliary_brakes_status_enum#BSMStoreSignal.Veh1BSM.vehicle_height_cm#BSMStoreSignal.Veh1BSM.vehicle_width_cm
  wires:
  BSM Data/1 -> Bus Selector/1
  Bus Selector/31 -> Data Store Write/31  "<value (signal 31)>"
  Bus Selector/10 -> Data Store Write/10  "<value (signal 10)>"
  Bus Selector/8 -> Data Store Write/8  "<value (signal 8)>"
  Bus Selector/13 -> Data Store Write/13  "<value (signal 13)>"
  Bus Selector/11 -> Data Store Write/11  "<value (signal 11)>"
  Bus Selector/12 -> Data Store Write/12  "<value (signal 12)>"
  Bus Selector/19 -> Data Store Write/19  "<signal19 (signal 19)>"
  Bus Selector/20 -> Data Store Write/20  "<signal20 (signal 20)>"
  Bus Selector/18 -> Data Store Write/18  "<signal18 (signal 18)>"
  Bus Selector/14 -> Data Store Write/14  "<value (signal 14)>"
  Bus Selector/22 -> Data Store Write/22  "<signal22 (signal 22)>"
  Bus Selector/44 -> Data Store Write/44  "<signal44 (signal 44)>"
  Bus Selector/42 -> Data Store Write/42  "<signal42 (signal 42)>"
  Bus Selector/35 -> Data Store Write/35  "<value (signal 35)>"
  Bus Selector/36 -> Data Store Write/36  "<signal36 (signal 36)>"
  Bus Selector/45 -> Data Store Write/45  "<signal45 (signal 45)>"
  Bus Selector/7 -> Data Store Write/7  "<value (signal 7)>"
  Bus Selector/39 -> Data Store Write/39  "<signal39 (signal 39)>"
  Bus Selector/23 -> Data Store Write/23  "<signal23 (signal 23)>"
  Bus Selector/43 -> Data Store Write/43  "<signal43 (signal 43)>"
  Bus Selector/28 -> Data Store Write/28  "<signal28 (signal 28)>"
  Bus Selector/29 -> Data Store Write/29  "<value (signal 29)>"
  Bus Selector/25 -> Data Store Write/25  "<signal25 (signal 25)>"
  Bus Selector/30 -> Data Store Write/30  "<signal30 (signal 30)>"
  Bus Selector/32 -> Data Store Write/32  "<signal32 (signal 32)>"
  Bus Selector/27 -> Data Store Write/27  "<value (signal 27)>"
  Bus Selector/26 -> Data Store Write/26  "<value (signal 26)>"
  Bus Selector/24 -> Data Store Write/24  "<signal24 (signal 24)>"
  Bus Selector/16 -> Data Store Write/16  "<signal16 (signal 16)>"
  Bus Selector/33 -> Data Store Write/33  "<signal33 (signal 33)>"
  Bus Selector/17 -> Data Store Write/17  "<signal17 (signal 17)>"
  Bus Selector/15 -> Data Store Write/15  "<value (signal 15)>"
  Bus Selector/41 -> Data Store Write/41  "<signal41 (signal 41)>"
  Bus Selector/37 -> Data Store Write/37  "<signal37 (signal 37)>"
  Bus Selector/9 -> Data Store Write/9  "<value (signal 9)>"
  Bus Selector/3 -> Data Store Write/3  "<value (signal 3)>"
  Bus Selector/38 -> Data Store Write/38  "<signal38 (signal 38)>"
  Bus Selector/5 -> Data Store Write/5  "<signal5 (signal 5)>"
  Bus Selector/4 -> Data Store Write/4  "<signal4 (signal 4)>"
  Bus Selector/1 -> Data Store Write/1  "<signal1 (signal 1)>"
  Bus Selector/40 -> Data Store Write/40  "<signal40 (signal 40)>"
  Bus Selector/2 -> Data Store Write/2  "<value (signal 2)>"
  Bus Selector/34 -> Data Store Write/34  "<value (signal 34)>"
  Bus Selector/21 -> Data Store Write/21  "<signal21 (signal 21)>"
  Bus Selector/6 -> Data Store Write/6  "<signal6 (signal 6)>"

== system dsrc_transmitter/BSM Broadcast/Write TORC Data/Veh 2 Data Update ==
  BSM Data : Inport
  Action Port : ActionPort
  Bus Selector : BusSelector  OutputSignals=signal1 (signal 1),value (signal 2),value (signal 3),signal4 (signal 4),signal5 (signal 5),signal6 (signal 6),value (signal 7),value (signal 8),value (signal 9),value (signal 10),value (signal 11),value (signal 12),value (signal 13),value (signal 14),value (signal 15),signal16 (signal 16),signal17 (signal 17),signal18 (signal 18),signal19 (signal 19),signal20 (signal 20),signal21 (signal 21),signal22 (signal 22),signal23 (signal 23),signal24 (signal 24),signal25 (signal 25),value (signal 26),value (signal 27),signal28 (signal 28),value (signal 29),signal30 (signal 30),value (signal 31),signal32 (signal 32),signal33 (signal 33),value (signal 34),value (signal 35),signal36 (signal 36),signal37 (signal 37),signal38 (signal 38),signal39 (signal 39),signal40 (signal 40),signal41 (signal 41),signal42 (signal 42),signal43 (signal 43),signal44 (signal 44),signal45 (signal 45)
  Data Store Write1 : DataStoreWrite  DataStoreName=BSMStoreSignal  DataStoreElements=BSMStoreSignal.Veh2BSM.caccFlags_bitmask#BSMStoreSignal.Veh2BSM.setSpeed_m_s#BSMStoreSignal.Veh2BSM.throtPos_percent#BSMStoreSignal.Veh2BSM.lclPN_mm#BSMStoreSignal.Veh2BSM.lclPE_mm#BSMStoreSignal.Veh2BSM.lclPD_mm#BSMStoreSignal.Veh2BSM.roll_deg#BSMStoreSignal.Veh2BSM.pitch_deg#BSMStoreSignal.Veh2BSM.yaw_deg#BSMStoreSignal.Veh2BSM.hPosAcry_m#BSMStoreSignal.Veh2BSM.vPosAcry_m#BSMStoreSignal.Veh2BSM.frwdVel_m_s#BSMStoreSignal.Veh2BSM.rightVel_m_s#BSMStoreSignal.Veh2BSM.downVel_m_s#BSMStoreSignal.Veh2BSM.velAcc_m_s#BSMStoreSignal.Veh2BSM.frwdAcc_mm_s_s#BSMStoreSignal.Veh2BSM.rightAcc_mm_s_s#BSMStoreSignal.Veh2BSM.dwnAcc_mm_s_s#BSMStoreSignal.Veh2BSM.msgID#BSMStoreSignal.Veh2BSM.msgCnt#BSMStoreSignal.Veh2BSM.id#BSMStoreSignal.Veh2BSM.secMark_ms#BSMStoreSignal.Veh2BSM.lat_deg#BSMStoreSignal.Veh2BSM.lon_deg#BSMStoreSignal.Veh2BSM.elev_m#BSMStoreSignal.Veh2BSM.semi_major_accuracy_m#BSMStoreSignal.Veh2BSM.semi_minor_accuracy_m#BSMStoreSignal.Veh2BSM.semi_major_accuracy_orientation_deg#BSMStoreSignal.Veh2BSM.speed_m_s#BSMStoreSignal.Veh2BSM.transmission_enum#BSMStoreSignal.Veh2BSM.heading_deg#BSMStoreSignal.Veh2BSM.angle_deg#BSMStoreSignal.Veh2BSM.vertical_acceleration_g#BSMStoreSignal.Veh2BSM.lat_acceleration_m_s_s#BSMStoreSignal.Veh2BSM.long_acceleration_m_s_s#BSMStoreSignal.Veh2BSM.yaw_rate_deg_s#BSMStoreSignal.Veh2BSM.wheelBrakes_bitmask#BSMStoreSignal.Veh2BSM.wheelBrakesUnavailable#BSMStoreSignal.Veh2BSM.tractionControlState_enum#BSMStoreSignal.Veh2BSM.anti_lock_brake_status_enum#BSMStoreSignal.Veh2BSM.stability_control_status_enum#BSMStoreSignal.Veh2BSM.brake_boost_enum#BSMStoreSignal.Veh2BSM.auxiliary_brakes_status_enum#BSMStoreSignal.Veh2BSM.vehicle_height_cm#BSMStoreSignal.Veh2BSM.vehicle_width_cm
  wires:
  BSM Data/1 -> Bus Selector/1
  Bus Selector/31 -> Data Store Write1/31  "<value (signal 31)>"
  Bus Selector/10 -> Data Store Write1/10  "<value (signal 10)>"
  Bus Selector/8 -> Data Store Write1/8  "<value (signal 8)>"
  Bus Selector/13 -> Data Store Write1/13  "<value (signal 13)>"
  Bus Selector/11 -> Data Store Write1/11  "<value (signal 11)>"
  Bus Selector/12 -> Data Store Write1/12  "<value (signal 12)>"
  Bus Selector/19 -> Data Store Write1/19  "<signal19 (signal 19)>"
  Bus Selector/20 -> Data Store Write1/20  "<signal20 (signal 20)>"
  Bus Selector/18 -> Data Store Write1/18  "<signal18 (signal 18)>"
  Bus Selector/14 -> Data Store Write1/14  "<value (signal 14)>"
  Bus Selector/22 -> Data Store Write1/22  "<signal22 (signal 22)>"
  Bus Selector/44 -> Data Store Write1/44  "<signal44 (signal 44)>"
  Bus Selector/42 -> Data Store Write1/42  "<signal42 (signal 42)>"
  Bus Selector/35 -> Data Store Write1/35  "<value (signal 35)>"
  Bus Selector/36 -> Data Store Write1/36  "<signal36 (signal 36)>"
  Bus Selector/45 -> Data Store Write1/45  "<signal45 (signal 45)>"
  Bus Selector/7 -> Data Store Write1/7  "<value (signal 7)>"
  Bus Selector/39 -> Data Store Write1/39  "<signal39 (signal 39)>"
  Bus Selector/23 -> Data Store Write1/23  "<signal23 (signal 23)>"
  Bus Selector/43 -> Data Store Write1/43  "<signal43 (signal 43)>"
  Bus Selector/28 -> Data Store Write1/28  "<signal28 (signal 28)>"
  Bus Selector/29 -> Data Store Write1/29  "<value (signal 29)>"
  Bus Selector/25 -> Data Store Write1/25  "<signal25 (signal 25)>"
  Bus Selector/30 -> Data Store Write1/30  "<signal30 (signal 30)>"
  Bus Selector/32 -> Data Store Write1/32  "<signal32 (signal 32)>"
  Bus Selector/27 -> Data Store Write1/27  "<value (signal 27)>"
  Bus Selector/26 -> Data Store Write1/26  "<value (signal 26)>"
  Bus Selector/24 -> Data Store Write1/24  "<signal24 (signal 24)>"
  Bus Selector/16 -> Data Store Write1/16  "<signal16 (signal 16)>"
  Bus Selector/33 -> Data Store Write1/33  "<signal33 (signal 33)>"
  Bus Selector/17 -> Data Store Write1/17  "<signal17 (signal 17)>"
  Bus Selector/15 -> Data Store Write1/15  "<value (signal 15)>"
  Bus Selector/41 -> Data Store Write1/41  "<signal41 (signal 41)>"
  Bus Selector/37 -> Data Store Write1/37  "<signal37 (signal 37)>"
  Bus Selector/9 -> Data Store Write1/9  "<value (signal 9)>"
  Bus Selector/3 -> Data Store Write1/3  "<value (signal 3)>"
  Bus Selector/38 -> Data Store Write1/38  "<signal38 (signal 38)>"
  Bus Selector/5 -> Data Store Write1/5  "<signal5 (signal 5)>"
  Bus Selector/4 -> Data Store Write1/4  "<signal4 (signal 4)>"
  Bus Selector/1 -> Data Store Write1/1  "<signal1 (signal 1)>"
  Bus Selector/40 -> Data Store Write1/40  "<signal40 (signal 40)>"
  Bus Selector/2 -> Data Store Write1/2  "<value (signal 2)>"
  Bus Selector/34 -> Data Store Write1/34  "<value (signal 34)>"
  Bus Selector/21 -> Data Store Write1/21  "<signal21 (signal 21)>"
  Bus Selector/6 -> Data Store Write1/6  "<signal6 (signal 6)>"
